simulink model "topology_comparison_eff"  (R2024b)
settings: Solver=ode23tb  StartTime=0.0  StopTime=4  MaxStep=1e-4  MinStep=1e-9  RelTol=1e-3
InitFcn:
  | sw_freq=60e3;
  | eff_rms_freq=sw_freq/10;
  | V_high=80;
  | 
  | L_ind=300e-6;
  | L_res=20e-3;
  | 
  | MOS_Ron=10e-3;
  | MOS_Vfw=1.2;
  | 
  | DIO_Vfw=0.9;
  | DIO_Ron=2e-3;
  | 
  | TRC_Res=5e-3;
  | 
  | sync_mode=1;
  | 
  | buck_p=0.02;
  | buck_i=0.8;
  | 
  | inter_bdc_p=0.02;
  | inter_bdc_i=0.9;
  | 
  | asym_bdc_p=0.02;
  | asym_bdc_i=1.1;
values from neighbouring files (symbols this model uses):
  runtime = 4    [compare_conv_eff.m]
  timestep = runtime/size(curr_range,2)    [compare_conv_eff.m]
undefined symbols (not defined in the file or in its folder): V_low
libraries: spsMeanLib x14, spsGroundLib x14, spsSeriesRLCBranchLib x14, spsMosfetLib x10, slpidlib x7, spsDCVoltageSourceLib x6, spsMultimeterLib x3, spsDiodeLib x2, embmathops x1, spsStairGeneratorLib x1, spspowerguiLib x1
(part 1 of 2)
settings Model: SimulationMode=rapid-accelerator  Creator=adamo  LastModifiedBy=adamo
settings DebuggingCC: MaskedZcDiagnostic=none  IgnoredZcDiagnostic=none
settings HardwareCC: ProdHWDeviceType=AMD->x86-64 (Windows64)
settings RTWCC: BuildConfiguration=Faster Runs  CheckMdlBeforeBuild=Error
settings GRTTargetCC: OptimizeReductions=on
settings SimscapeCC: SimscapeCompileComponentReuse=on  SimscapeCompileArtifactsDiskCache=on

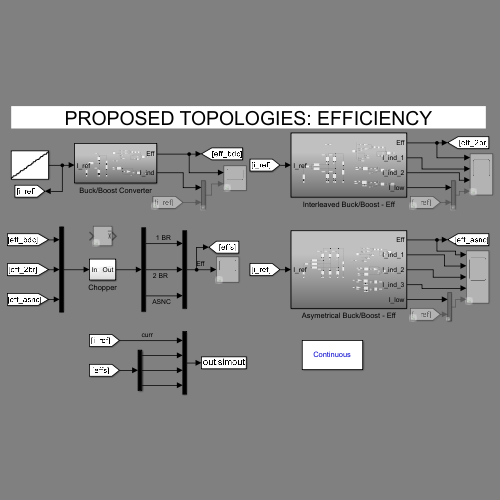
[thumbnail: Simulink's stored preview of the top-level diagram]
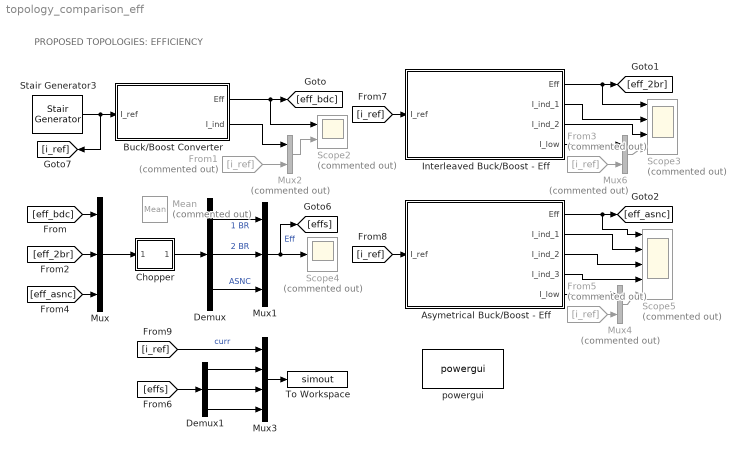
== system topology_comparison_eff ==
  note: PROPOSED TOPOLOGIES: EFFICIENCY
  Asymetrical Buck/Boost - Eff : Subsystem
  Buck/Boost Converter : Subsystem
  Chopper : Subsystem
  Demux : Demux  Outputs=3
  Demux1 : Demux  Outputs=3
  From1 : From  Commented=on  GotoTag=i_ref
  From3 : From  Commented=on  GotoTag=i_ref
  From5 : From  Commented=on  GotoTag=i_ref
  Interleaved Buck/Boost - Eff : Subsystem
  Mean : spsMeanLib/Mean  Commented=on  Freq=sw_freq/10  Vinit=0  Ts=0
  Mux : Mux  Inputs=3
  Mux1 : Mux  Inputs=3
  Mux2 : Mux  Commented=on  Inputs=2
  Mux3 : Mux
  Mux4 : Mux  Commented=on  Inputs=2
  Mux6 : Mux  Commented=on  Inputs=2
  Scope2 : Scope  Commented=on  NumInputPorts=2
  Scope3 : Scope  Commented=on  NumInputPorts=4
  Scope4 : Scope  Commented=on
  Scope5 : Scope  Commented=on  NumInputPorts=5
  Stair Generator3 : spsStairGeneratorLib/Stair Generator  t=[0:timestep:runtime-timestep]  e=curr_range  Ts=0
  To Workspace : ToWorkspace  VariableName=simout  SampleTime=-1
  powergui : spspowerguiLib/powergui  Priority=1  SimulationMode=Continuous  SampleTime=50e-6  frequency=60  Iterations=50  frequencyindice=0  Pbase=100e6  ErrMax=1e-4  UnitsV=kV  UnitsW=MW  buscounter=0  FunctionMessages=off  echomessages=off  EnableUseOfTLC=off  CurrentSourceSwitches=off  DisableSnubberDevices=on  DisableRonSwitches=off  DisableVfSwitches=off  DisplayEquations=off  AutomaticDiscreteSolvers=off  SolverType=Tustin/Backward Euler (TBE)  Interpol=off  ExternalGateDelay=off  methode=on  Ts=100  x0status=blocks  SPID=on  SwTol=0  HookPort=off  NonlinearTolerance=1e-4  nMaxIteration=100  ContinueOnMaxIteration=off  RestoreLinks=warning  ResistiveCurrentMeasurement=off  Frange=[0:2:500]  Ylog=off  Xlog=on  ShowGrid=off  save=off  variable=ZData  structure=0  ZoomFFT=off  StartTime=0.0  cycles=1  DisplayStyle=1  fundamental=60  FreqAxis=off  MaxFrequency=1000  frequencyindicesteady=1  RmsSteady=1  display=off
  wires:
  Stair Generator3/1 -> [i_ref], Buck/Boost Converter/1(I_ref)
  [i_ref] -> Interleaved Buck/Boost - Eff/1(I_ref)
  [i_ref] -> Asymetrical Buck/Boost - Eff/1(I_ref)
  Buck/Boost Converter/2(I_ind) -> Mux2/1
  Interleaved Buck/Boost - Eff/1(Eff) -> Scope3/1, [eff_2br]
  Interleaved Buck/Boost - Eff/3(I_ind_2) -> Scope3/3
  Interleaved Buck/Boost - Eff/2(I_ind_1) -> Scope3/2
  Asymetrical Buck/Boost - Eff/3(I_ind_2) -> Scope5/3
  Asymetrical Buck/Boost - Eff/4(I_ind_3) -> Scope5/4
  Buck/Boost Converter/1(Eff) -> Scope2/1, [eff_bdc]
  Asymetrical Buck/Boost - Eff/1(Eff) -> Scope5/1, [eff_asnc]
  [eff_bdc] -> Mux/1
  [eff_2br] -> Mux/2
  [eff_asnc] -> Mux/3
  Mux/1 -> Chopper/1(In1)
  Chopper/1(Out1) -> Demux/1
  Demux/1 -> Mux1/1  "1 BR"
  Demux/2 -> Mux1/2  "2 BR"
  Demux/3 -> Mux1/3  "ASNC"
  Mux1/1 -> [effs], Scope4/1  "Eff"
  [i_ref] -> Mux3/1  "curr"
  Mux3/1 -> To Workspace/1
  [effs] -> Demux1/1
  Demux1/1 -> Mux3/2
  Demux1/2 -> Mux3/3
  Demux1/3 -> Mux3/4
  Interleaved Buck/Boost - Eff/4(I_low) -> Mux6/1
  Asymetrical Buck/Boost - Eff/2(I_ind_1) -> Scope5/2
  From1/1 -> Mux2/2
  Mux2/1 -> Scope2/2
  From3/1 -> Mux6/2
  Mux6/1 -> Scope3/4
  From5/1 -> Mux4/2
  Asymetrical Buck/Boost - Eff/5(I_low) -> Mux4/1
  Mux4/1 -> Scope5/5

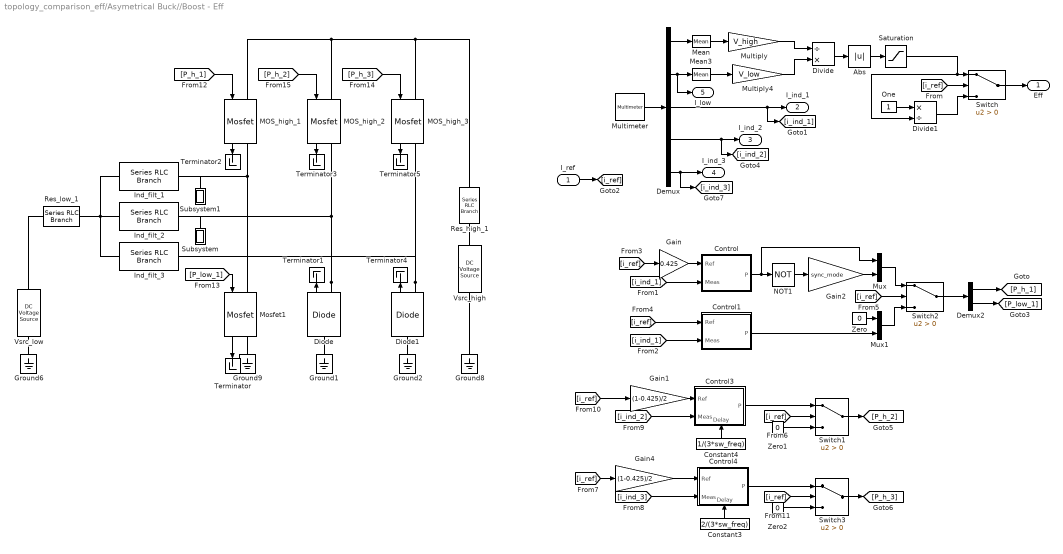
== system topology_comparison_eff/Asymetrical Buck//Boost - Eff ==
  I_ref : Inport
  Abs : Abs  SaturateOnIntegerOverflow=off
  Constant3 : Constant  Value=2/(3*sw_freq)
  Constant4 : Constant  Value=1/(3*sw_freq)
  Control : Subsystem
  Control1 : Subsystem
  Control3 : Subsystem
      settings: PortSchema="{\"entries\":[{\"content\":{\"sides\":[{\"content\":{\"connectorIds\":[\"In1\",\"In2\"]},\"type\":\"ConnectorPlacement.EquallySpacedRectSide\",\"uuid\":\"44975c06-6cb3-4b92-aa2e-c11b859d13e4\"},{\"content\":{\"connectorIds\":[\"Out1\"],\"side\":\"RIGHT\"},\"type\":\"ConnectorPlacement.EquallySpacedRectSide\",\"uuid\":\"ebdc9065-5b19-4aa7-8841-916fd82a5d31\"},{\"content\":{\"side\":\"TOP\"},\"type\":\"ConnectorPlacement.EquallySpacedRectSide\",\"uuid\":\"027925ea-888b-4bcf-b8a4-44694d0e275e\"},{\"content\":{\"connectorIds\":[\"In3\"],\"side\":\"BOTTOM\"},\"type\":\"ConnectorPlacement.EquallySpacedRectSide\",\"uuid\":\"415fb0af-dd9a-4309-9118-76332ed11379\"}]},\"type\":\"ConnectorPlacement.EquallySpacedConnector\",\"uuid\":\"3cd19595-535e-42c3-a0e6-40045bedee28\"}],\"packageUris\":[\"http://schema.mathworks.com/mf0/Connector/R2020b\"],\"version\":\"1.0\"}"
  Control4 : Subsystem
      settings: PortSchema="{\"entries\":[{\"content\":{\"sides\":[{\"content\":{\"connectorIds\":[\"In1\",\"In2\"]},\"type\":\"ConnectorPlacement.EquallySpacedRectSide\",\"uuid\":\"44975c06-6cb3-4b92-aa2e-c11b859d13e4\"},{\"content\":{\"connectorIds\":[\"Out1\"],\"side\":\"RIGHT\"},\"type\":\"ConnectorPlacement.EquallySpacedRectSide\",\"uuid\":\"ebdc9065-5b19-4aa7-8841-916fd82a5d31\"},{\"content\":{\"side\":\"TOP\"},\"type\":\"ConnectorPlacement.EquallySpacedRectSide\",\"uuid\":\"027925ea-888b-4bcf-b8a4-44694d0e275e\"},{\"content\":{\"connectorIds\":[\"In3\"],\"side\":\"BOTTOM\"},\"type\":\"ConnectorPlacement.EquallySpacedRectSide\",\"uuid\":\"9488b47a-c58c-42e9-bacd-7bb9f563b775\"}]},\"type\":\"ConnectorPlacement.EquallySpacedConnector\",\"uuid\":\"3cd19595-535e-42c3-a0e6-40045bedee28\"}],\"packageUris\":[\"http://schema.mathworks.com/mf0/Connector/R2020b\"],\"version\":\"1.0\"}"
  Demux : Demux  Outputs=5
  Demux2 : Demux  Outputs=2
  Diode : spsDiodeLib/Diode  Ron=DIO_Ron  Lon=0  Vf=DIO_Vfw  IC=0  UseSnubber=0  Rs=500  Cs=250e-9  Measurements=on
  Diode1 : spsDiodeLib/Diode  Ron=DIO_Ron  Lon=0  Vf=DIO_Vfw  IC=0  UseSnubber=0  Rs=500  Cs=250e-9  Measurements=on
  Divide : Product  Inputs=/*
  Divide1 : Product  Inputs=*/
  Gain : Gain  Gain=0.425
  Gain1 : Gain  Gain=(1-0.425)/2
  Gain2 : Gain  Gain=sync_mode  OutDataTypeStr=double
  Gain4 : Gain  Gain=(1-0.425)/2
  Ground{1..2,6,8..9} (5 alike) : spsGroundLib/Ground  LConnTagsString=a
  Ind_filt_1 : spsSeriesRLCBranchLib/Series RLC Branch  LConnTagsString=__new0  RConnTagsString=__new0  BranchType=RL  Resistance=L_res  Inductance=L_ind  SetiL0=off  InitialCurrent=0  Capacitance=1e-6  Setx0=off  InitialVoltage=0  Measurements=Branch current
  Ind_filt_2 : spsSeriesRLCBranchLib/Series RLC Branch  LConnTagsString=__new0  RConnTagsString=__new0  BranchType=RL  Resistance=L_res  Inductance=L_ind  SetiL0=off  InitialCurrent=0  Capacitance=1e-6  Setx0=off  InitialVoltage=0  Measurements=Branch current
  Ind_filt_3 : spsSeriesRLCBranchLib/Series RLC Branch  LConnTagsString=__new0  RConnTagsString=__new0  BranchType=RL  Resistance=L_res  Inductance=L_ind  SetiL0=off  InitialCurrent=0  Capacitance=1e-6  Setx0=off  InitialVoltage=0  Measurements=Branch current
  MOS_high_1 : spsMosfetLib/Mosfet  Ron=MOS_Ron  Lon=0  Rd=DIO_Ron  Vfd=MOS_Vfw  IC=0  Rs=1e5  Cs=inf  Measurements=on
  MOS_high_2 : spsMosfetLib/Mosfet  Ron=MOS_Ron  Lon=0  Rd=DIO_Ron  Vfd=MOS_Vfw  IC=0  Rs=1e5  Cs=inf  Measurements=on
  MOS_high_3 : spsMosfetLib/Mosfet  Ron=MOS_Ron  Lon=0  Rd=DIO_Ron  Vfd=MOS_Vfw  IC=0  Rs=1e5  Cs=inf  Measurements=on
  Mean : spsMeanLib/Mean  Freq=eff_rms_freq  Vinit=1  Ts=0
  Mean3 : spsMeanLib/Mean  Freq=eff_rms_freq  Vinit=1  Ts=0
  Mosfet1 : spsMosfetLib/Mosfet  Ron=MOS_Ron  Lon=0  Rd=DIO_Ron  Vfd=MOS_Vfw  IC=0  Rs=1e5  Cs=inf  Measurements=on
  Multimeter : spsMultimeterLib/Multimeter  L=12  sel=[4 5 1 2 3]  yselected={}  Gain=[1 1 1 1 1]  OutputType=Complex  PlotAtSimulationStop=off  PhasorSimulation=off
  Multiply : Gain  Gain=V_high
  Multiply4 : Gain  Gain=V_low
  Mux : Mux  Inputs=2
  Mux1 : Mux  Inputs=2
  NOT1 : Logic  Operator=NOT  IconShape=distinctive  AllPortsSameDT=off  OutDataTypeStr=boolean
  One : Constant  OutDataTypeStr=Inherit: Inherit via back propagation
  Res_high_1 : spsSeriesRLCBranchLib/Series RLC Branch  LConnTagsString=__new0  RConnTagsString=__new0  BranchType=R  Resistance=TRC_Res  Inductance=1e-3  SetiL0=off  InitialCurrent=0  Capacitance=1e-6  Setx0=off  InitialVoltage=0  Measurements=Branch current
  Res_low_1 : spsSeriesRLCBranchLib/Series RLC Branch  LConnTagsString=__new0  RConnTagsString=__new0  BranchType=R  Resistance=TRC_Res  Inductance=1e-3  SetiL0=off  InitialCurrent=0  Capacitance=1e-6  Setx0=off  InitialVoltage=0  Measurements=Branch current
  Saturation : Saturate  UpperLimit=0.9999  LowerLimit=0.4
  Subsystem : Subsystem
      settings: PortSchema="{\"entries\":[{\"content\":{\"sides\":[{\"content\":{},\"type\":\"ConnectorPlacement.EquallySpacedRectSide\",\"uuid\":\"333a472d-5660-403e-9749-9e5a485a4e51\"},{\"content\":{\"side\":\"RIGHT\"},\"type\":\"ConnectorPlacement.EquallySpacedRectSide\",\"uuid\":\"46e3a3df-9b43-4056-bf49-6d97e0ff375e\"},{\"content\":{\"connectorIds\":[\"LConn1\"],\"side\":\"TOP\"},\"type\":\"ConnectorPlacement.EquallySpacedRectSide\",\"uuid\":\"a9be43b9-3284-437d-b483-2a714199e3a2\"}]},\"type\":\"ConnectorPlacement.EquallySpacedConnector\",\"uuid\":\"6030dd83-63ea-4a67-9f73-95d000b3af89\"}],\"packageUris\":[\"http://schema.mathworks.com/mf0/Connector/R2020b\"],\"version\":\"1.0\"}"
  Subsystem1 : Subsystem
      settings: PortSchema="{\"entries\":[{\"content\":{\"sides\":[{\"content\":{},\"type\":\"ConnectorPlacement.EquallySpacedRectSide\",\"uuid\":\"333a472d-5660-403e-9749-9e5a485a4e51\"},{\"content\":{\"side\":\"RIGHT\"},\"type\":\"ConnectorPlacement.EquallySpacedRectSide\",\"uuid\":\"46e3a3df-9b43-4056-bf49-6d97e0ff375e\"},{\"content\":{\"connectorIds\":[\"LConn1\"],\"side\":\"TOP\"},\"type\":\"ConnectorPlacement.EquallySpacedRectSide\",\"uuid\":\"a9be43b9-3284-437d-b483-2a714199e3a2\"}]},\"type\":\"ConnectorPlacement.EquallySpacedConnector\",\"uuid\":\"6030dd83-63ea-4a67-9f73-95d000b3af89\"}],\"packageUris\":[\"http://schema.mathworks.com/mf0/Connector/R2020b\"],\"version\":\"1.0\"}"
  Switch{,1..3} (4 alike) : Switch  Criteria=u2 > Threshold  SaturateOnIntegerOverflow=off  InputSameDT=off
  Terminator{,1..5} (6 alike) : Terminator
  Vsrc_high : spsDCVoltageSourceLib/DC Voltage Source  Amplitude=V_high  Measurements=None
  Vsrc_low : spsDCVoltageSourceLib/DC Voltage Source  Amplitude=V_low  Measurements=None
  Zero : Constant  Value=0  OutDataTypeStr=Inherit: Inherit via back propagation
  Zero1 : Constant  Value=0  OutDataTypeStr=Inherit: Inherit via back propagation
  Zero2 : Constant  Value=0  OutDataTypeStr=Inherit: Inherit via back propagation
  Eff : Outport
  I_ind_1 : Outport  Port=2
  I_ind_2 : Outport  Port=3
  I_ind_3 : Outport  Port=4
  I_low : Outport  Port=5
  wires:
  [P_h_1] -> MOS_high_1/1
  MOS_high_1/1 -> Terminator2/1
  Mosfet1/1 -> Terminator/1
  [P_low_1] -> Mosfet1/1
  Diode/1 -> Terminator1/1
  MOS_high_2/1 -> Terminator3/1
  Diode1/1 -> Terminator4/1
  MOS_high_3/1 -> Terminator5/1
  [P_h_3] -> MOS_high_3/1
  Multimeter/1 -> Demux/1
  One/1 -> Divide1/1
  Mean/1 -> Multiply/1
  Divide1/1 -> Switch/3
  Saturation/1 -> Divide1/2, Switch/1
  Divide/1 -> Abs/1
  Switch/1 -> Eff/1
  Abs/1 -> Saturation/1
  Control/1(P) -> Mux/1, NOT1/1
  [i_ref] -> Gain/1
  Switch2/1 -> Demux2/1
  Mux/1 -> Switch2/1
  [i_ind_1] -> Control/2(Meas)
  Demux2/2 -> [P_low_1]
  Demux2/1 -> [P_h_1]
  Gain2/1 -> Mux/2
  [i_ref] -> Switch2/2
  I_ref/1 -> [i_ref]
  [i_ref] -> Switch/2
  NOT1/1 -> Gain2/1
  [P_h_2] -> MOS_high_2/1
  Gain/1 -> Control/1(Ref)
  [i_ref] -> Control1/1(Ref)
  [i_ind_1] -> Control1/2(Meas)
  Control1/1(P) -> Mux1/2
  Mean3/1 -> Multiply4/1
  Demux/1 -> Mean/1
  Demux/2 -> I_low/1, Mean3/1
  Demux/5 -> [i_ind_3], I_ind_3/1
  Demux/4 -> [i_ind_2], I_ind_2/1
  Demux/3 -> I_ind_1/1, [i_ind_1]
  Multiply4/1 -> Divide/2
  Multiply/1 -> Divide/1
  Mux1/1 -> Switch2/3
  Zero/1 -> Mux1/1
  Constant4/1 -> Control3/3(Delay)
  Constant3/1 -> Control4/3(Delay)
  [i_ref] -> Gain1/1
  Gain1/1 -> Control3/1(Ref)
  [i_ind_2] -> Control3/2(Meas)
  Control3/1(P) -> Switch1/1
  Switch1/1 -> [P_h_2]
  Zero1/1 -> Switch1/3
  [i_ref] -> Switch1/2
  [i_ind_3] -> Control4/2(Meas)
  [i_ref] -> Gain4/1
  Gain4/1 -> Control4/1(Ref)
  [i_ref] -> Switch3/2
  Control4/1(P) -> Switch3/1
  Switch3/1 -> [P_h_3]
  Zero2/1 -> Switch3/3
  connections:
  Diode/RConn1 -- Ind_filt_2/LConn1 -- Subsystem/LConn1 -- MOS_high_2/RConn1
  MOS_high_1/RConn1 -- Subsystem1/LConn1 -- Ind_filt_1/LConn1 -- Mosfet1/LConn1
  Ground8/LConn1 -- Vsrc_high/LConn1
  Mosfet1/RConn1 -- Ground9/LConn1
  Ground6/LConn1 -- Vsrc_low/LConn1
  Diode/LConn1 -- Ground1/LConn1
  Diode1/RConn1 -- Ind_filt_3/LConn1 -- MOS_high_3/RConn1
  Diode1/LConn1 -- Ground2/LConn1
  Res_low_1/RConn1 -- Vsrc_low/RConn1
  Res_high_1/LConn1 -- Vsrc_high/RConn1
  Ind_filt_2/RConn1 -- Res_low_1/LConn1 -- Ind_filt_3/RConn1 -- Ind_filt_1/RConn1
  Res_high_1/RConn1 -- MOS_high_1/LConn1 -- MOS_high_2/LConn1 -- MOS_high_3/LConn1

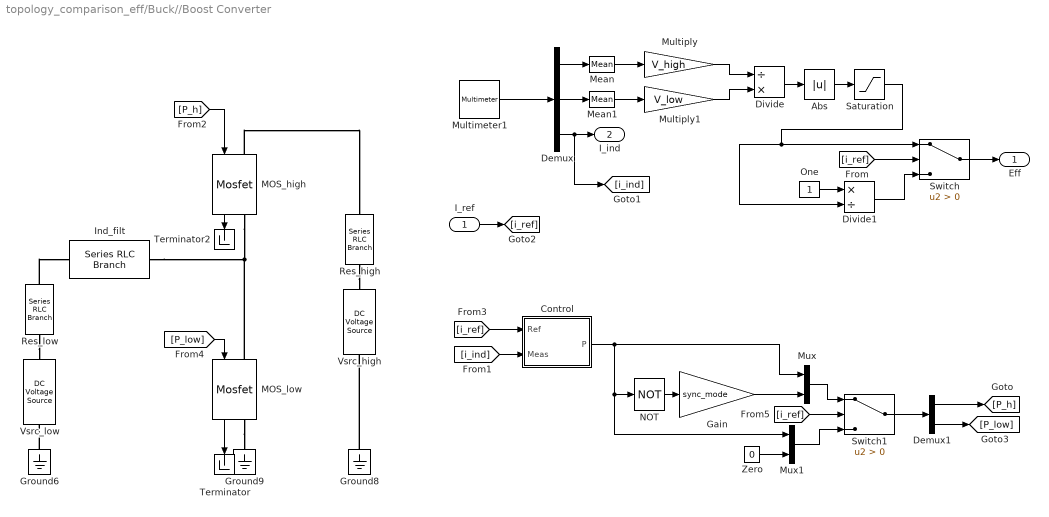
== system topology_comparison_eff/Buck//Boost Converter ==
  I_ref : Inport
  Abs : Abs  SaturateOnIntegerOverflow=off
  Control : Subsystem
  Demux : Demux  Outputs=3
  Demux1 : Demux  Outputs=2
  Divide : Product  Inputs=/*
  Divide1 : Product  Inputs=*/
  Gain : Gain  Gain=sync_mode  OutDataTypeStr=double
  Ground6 : spsGroundLib/Ground  LConnTagsString=a
  Ground8 : spsGroundLib/Ground  LConnTagsString=a
  Ground9 : spsGroundLib/Ground  LConnTagsString=a
  Ind_filt : spsSeriesRLCBranchLib/Series RLC Branch  LConnTagsString=__new0  RConnTagsString=__new0  BranchType=RL  Resistance=L_res  Inductance=L_ind  SetiL0=off  InitialCurrent=0  Capacitance=1e-6  Setx0=off  InitialVoltage=0  Measurements=Branch current
  MOS_high : spsMosfetLib/Mosfet  Ron=MOS_Ron  Lon=0  Rd=DIO_Ron  Vfd=MOS_Vfw  IC=0  Rs=1e5  Cs=inf  Measurements=on
  MOS_low : spsMosfetLib/Mosfet  Ron=MOS_Ron  Lon=0  Rd=DIO_Ron  Vfd=MOS_Vfw  IC=0  Rs=1e5  Cs=inf  Measurements=on
  Mean : spsMeanLib/Mean  Freq=eff_rms_freq  Vinit=1  Ts=0
  Mean1 : spsMeanLib/Mean  Freq=eff_rms_freq  Vinit=1  Ts=0
  Multimeter1 : spsMultimeterLib/Multimeter  L=12  sel=[7 8 6]  yselected={}  Gain=[1 1 1]  OutputType=Complex  PlotAtSimulationStop=off  PhasorSimulation=off
  Multiply : Gain  Gain=V_high
  Multiply1 : Gain  Gain=V_low
  Mux : Mux  Inputs=2
  Mux1 : Mux  Inputs=2
  NOT : Logic  Operator=NOT  IconShape=distinctive  AllPortsSameDT=off  OutDataTypeStr=boolean
  One : Constant  OutDataTypeStr=Inherit: Inherit via back propagation
  Res_high : spsSeriesRLCBranchLib/Series RLC Branch  LConnTagsString=__new0  RConnTagsString=__new0  BranchType=R  Resistance=TRC_Res  Inductance=1e-3  SetiL0=off  InitialCurrent=0  Capacitance=1e-6  Setx0=off  InitialVoltage=0  Measurements=Branch current
  Res_low : spsSeriesRLCBranchLib/Series RLC Branch  LConnTagsString=__new0  RConnTagsString=__new0  BranchType=R  Resistance=TRC_Res  Inductance=1e-3  SetiL0=off  InitialCurrent=0  Capacitance=1e-6  Setx0=off  InitialVoltage=0  Measurements=Branch current
  Saturation : Saturate  UpperLimit=0.9999  LowerLimit=0.4
  Switch : Switch  Criteria=u2 > Threshold  SaturateOnIntegerOverflow=off  InputSameDT=off
  Switch1 : Switch  Criteria=u2 > Threshold  SaturateOnIntegerOverflow=off  InputSameDT=off
  Terminator : Terminator
  Terminator2 : Terminator
  Vsrc_high : spsDCVoltageSourceLib/DC Voltage Source  Amplitude=V_high  Measurements=None
  Vsrc_low : spsDCVoltageSourceLib/DC Voltage Source  Amplitude=V_low  Measurements=None
  Zero : Constant  Value=0  OutDataTypeStr=Inherit: Inherit via back propagation
  Eff : Outport
  I_ind : Outport  Port=2
  wires:
  MOS_low/1 -> Terminator/1
  MOS_high/1 -> Terminator2/1
  [P_h] -> MOS_high/1
  [P_low] -> MOS_low/1
  Multiply/1 -> Divide/1
  Demux/1 -> Mean/1
  Saturation/1 -> Divide1/2, Switch/1
  Multiply1/1 -> Divide/2
  Mean/1 -> Multiply/1
  Multimeter1/1 -> Demux/1
  Demux/2 -> Mean1/1
  Mean1/1 -> Multiply1/1
  One/1 -> Divide1/1
  Divide1/1 -> Switch/3
  Switch/1 -> Eff/1
  Divide/1 -> Abs/1
  Demux/3 -> [i_ind], I_ind/1
  Control/1(P) -> Mux1/1, NOT/1, Mux/1
  I_ref/1 -> [i_ref]
  [i_ref] -> Switch/2
  [i_ind] -> Control/2(Meas)
  [i_ref] -> Control/1(Ref)
  NOT/1 -> Gain/1
  Abs/1 -> Saturation/1
  [i_ref] -> Switch1/2
  Mux/1 -> Switch1/1
  Switch1/1 -> Demux1/1
  Demux1/1 -> [P_h]
  Demux1/2 -> [P_low]
  Zero/1 -> Mux1/2
  Mux1/1 -> Switch1/3
  Gain/1 -> Mux/2
  connections:
  MOS_high/LConn1 -- Res_high/RConn1
  MOS_low/RConn1 -- Ground9/LConn1
  MOS_high/RConn1 -- Ind_filt/LConn1 -- MOS_low/LConn1
  Ground8/LConn1 -- Vsrc_high/LConn1
  Ground6/LConn1 -- Vsrc_low/LConn1
  Res_low/LConn1 -- Ind_filt/RConn1
  Res_high/LConn1 -- Vsrc_high/RConn1
  Res_low/RConn1 -- Vsrc_low/RConn1

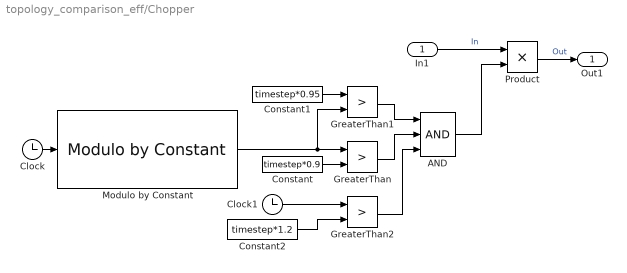
== system topology_comparison_eff/Chopper ==
  In1 : Inport
  AND : Logic  Inputs=3  IconShape=distinctive  AllPortsSameDT=off  OutDataTypeStr=boolean
  Clock : Clock
  Clock1 : Clock
  Constant : Constant  Value=timestep*0.9
  Constant1 : Constant  Value=timestep*0.95
  Constant2 : Constant  Value=timestep*1.2
  GreaterThan : RelationalOperator  Operator=>  OutDataTypeStr=boolean  RndMeth=Simplest  InputSameDT=off
  GreaterThan1 : RelationalOperator  Operator=>  OutDataTypeStr=boolean  RndMeth=Simplest  InputSameDT=off
  GreaterThan2 : RelationalOperator  Operator=>  OutDataTypeStr=boolean  RndMeth=Simplest  InputSameDT=off
  Modulo by Constant : embmathops/Modulo by Constant  Denominator=timestep  SimulateUsing=Code generation
  Product : Product
  Out1 : Outport
  wires:
  Clock/1 -> Modulo by Constant/1
  Constant/1 -> GreaterThan/2
  GreaterThan1/1 -> AND/1
  GreaterThan/1 -> AND/2
  AND/1 -> Product/2
  Modulo by Constant/1 -> GreaterThan1/2, GreaterThan/1
  Constant1/1 -> GreaterThan1/1
  In1/1 -> Product/1  "In"
  Product/1 -> Out1/1  "Out"
  Clock1/1 -> GreaterThan2/1
  GreaterThan2/1 -> AND/3
  Constant2/1 -> GreaterThan2/2

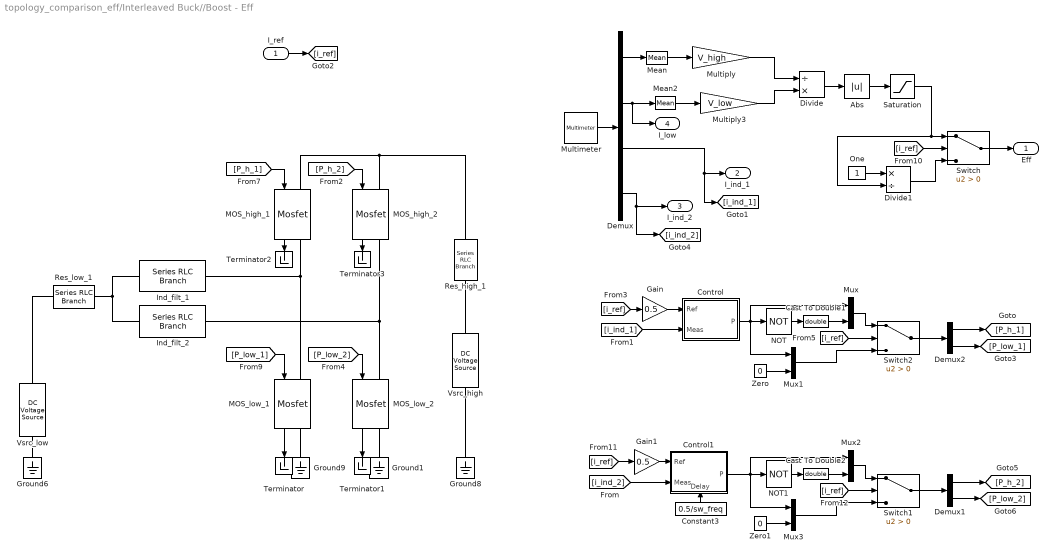
== system topology_comparison_eff/Interleaved Buck//Boost - Eff ==
  I_ref : Inport
  Abs : Abs  SaturateOnIntegerOverflow=off
  Cast To Double1 : DataTypeConversion  OutDataTypeStr=double  SaturateOnIntegerOverflow=off  RndMeth=Floor
  Cast To Double2 : DataTypeConversion  OutDataTypeStr=double  SaturateOnIntegerOverflow=off  RndMeth=Floor
  Constant3 : Constant  Value=0.5/sw_freq
  Control : Subsystem
  Control1 : Subsystem
      settings: PortSchema="{\"entries\":[{\"content\":{\"sides\":[{\"content\":{\"connectorIds\":[\"In1\",\"In2\"]},\"type\":\"ConnectorPlacement.EquallySpacedRectSide\",\"uuid\":\"44975c06-6cb3-4b92-aa2e-c11b859d13e4\"},{\"content\":{\"connectorIds\":[\"Out1\"],\"side\":\"RIGHT\"},\"type\":\"ConnectorPlacement.EquallySpacedRectSide\",\"uuid\":\"ebdc9065-5b19-4aa7-8841-916fd82a5d31\"},{\"content\":{\"side\":\"TOP\"},\"type\":\"ConnectorPlacement.EquallySpacedRectSide\",\"uuid\":\"027925ea-888b-4bcf-b8a4-44694d0e275e\"},{\"content\":{\"connectorIds\":[\"In3\"],\"side\":\"BOTTOM\"},\"type\":\"ConnectorPlacement.EquallySpacedRectSide\",\"uuid\":\"4b21ce2f-6f21-43cd-b77f-3dbeff0cb919\"}]},\"type\":\"ConnectorPlacement.EquallySpacedConnector\",\"uuid\":\"3cd19595-535e-42c3-a0e6-40045bedee28\"}],\"packageUris\":[\"http://schema.mathworks.com/mf0/Connector/R2020b\"],\"version\":\"1.0\"}"
  Demux : Demux
  Demux1 : Demux  Outputs=2
  Demux2 : Demux  Outputs=2
  Divide : Product  Inputs=/*
  Divide1 : Product  Inputs=*/
  Gain : Gain  Gain=0.5
  Gain1 : Gain  Gain=0.5
  Ground{1,6,8..9} (4 alike) : spsGroundLib/Ground  LConnTagsString=a
  Ind_filt_1 : spsSeriesRLCBranchLib/Series RLC Branch  LConnTagsString=__new0  RConnTagsString=__new0  BranchType=RL  Resistance=L_res*2/3  Inductance=L_ind  SetiL0=off  InitialCurrent=0  Capacitance=1e-6  Setx0=off  InitialVoltage=0  Measurements=Branch current
  Ind_filt_2 : spsSeriesRLCBranchLib/Series RLC Branch  LConnTagsString=__new0  RConnTagsString=__new0  BranchType=RL  Resistance=L_res*2/3  Inductance=L_ind  SetiL0=off  InitialCurrent=0  Capacitance=1e-6  Setx0=off  InitialVoltage=0  Measurements=Branch current
  MOS_high_1 : spsMosfetLib/Mosfet  Ron=MOS_Ron  Lon=0  Rd=DIO_Ron  Vfd=MOS_Vfw  IC=0  Rs=1e5  Cs=inf  Measurements=on
  MOS_high_2 : spsMosfetLib/Mosfet  Ron=MOS_Ron  Lon=0  Rd=DIO_Ron  Vfd=MOS_Vfw  IC=0  Rs=1e5  Cs=inf  Measurements=on
  MOS_low_1 : spsMosfetLib/Mosfet  Ron=MOS_Ron  Lon=0  Rd=DIO_Ron  Vfd=MOS_Vfw  IC=0  Rs=1e5  Cs=inf  Measurements=on
  MOS_low_2 : spsMosfetLib/Mosfet  Ron=MOS_Ron  Lon=0  Rd=DIO_Ron  Vfd=MOS_Vfw  IC=0  Rs=1e5  Cs=inf  Measurements=on
  Mean : spsMeanLib/Mean  Freq=eff_rms_freq  Vinit=1  Ts=0
  Mean2 : spsMeanLib/Mean  Freq=eff_rms_freq  Vinit=1  Ts=0
  Multimeter : spsMultimeterLib/Multimeter  L=12  sel=[11 12 9 10]  yselected={}  Gain=[1 1 1 1]  OutputType=Complex  PlotAtSimulationStop=off  PhasorSimulation=off
  Multiply : Gain  Gain=V_high
  Multiply3 : Gain  Gain=V_low
  Mux{,1..3} (4 alike) : Mux  Inputs=2
  NOT : Logic  Operator=NOT  IconShape=distinctive  AllPortsSameDT=off  OutDataTypeStr=boolean
  NOT1 : Logic  Operator=NOT  IconShape=distinctive  AllPortsSameDT=off  OutDataTypeStr=boolean
  One : Constant  OutDataTypeStr=Inherit: Inherit via back propagation
  Res_high_1 : spsSeriesRLCBranchLib/Series RLC Branch  LConnTagsString=__new0  RConnTagsString=__new0  BranchType=R  Resistance=TRC_Res  Inductance=1e-3  SetiL0=off  InitialCurrent=0  Capacitance=1e-6  Setx0=off  InitialVoltage=0  Measurements=Branch current
  Res_low_1 : spsSeriesRLCBranchLib/Series RLC Branch  LConnTagsString=__new0  RConnTagsString=__new0  BranchType=R  Resistance=TRC_Res  Inductance=1e-3  SetiL0=off  InitialCurrent=0  Capacitance=1e-6  Setx0=off  InitialVoltage=0  Measurements=Branch current
  Saturation : Saturate  UpperLimit=0.9999  LowerLimit=0.4
  Switch : Switch  Criteria=u2 > Threshold  SaturateOnIntegerOverflow=off  InputSameDT=off
  Switch1 : Switch  Criteria=u2 > Threshold  SaturateOnIntegerOverflow=off  InputSameDT=off
  Switch2 : Switch  Criteria=u2 > Threshold  SaturateOnIntegerOverflow=off  InputSameDT=off
  Terminator{,1..3} (4 alike) : Terminator
  Vsrc_high : spsDCVoltageSourceLib/DC Voltage Source  Amplitude=V_high  Measurements=None
  Vsrc_low : spsDCVoltageSourceLib/DC Voltage Source  Amplitude=V_low  Measurements=None
  Zero : Constant  Value=0  OutDataTypeStr=Inherit: Inherit via back propagation
  Zero1 : Constant  Value=0  OutDataTypeStr=Inherit: Inherit via back propagation
  Eff : Outport
  I_ind_1 : Outport  Port=2
  I_ind_2 : Outport  Port=3
  I_low : Outport  Port=4
  wires:
  [P_h_1] -> MOS_high_1/1
  [P_low_2] -> MOS_low_2/1
  MOS_high_1/1 -> Terminator2/1
  MOS_low_1/1 -> Terminator/1
  MOS_low_2/1 -> Terminator1/1
  MOS_high_2/1 -> Terminator3/1
  [P_low_1] -> MOS_low_1/1
  Divide/1 -> Abs/1
  Saturation/1 -> Divide1/2, Switch/1
  Divide1/1 -> Switch/3
  One/1 -> Divide1/1
  Multimeter/1 -> Demux/1
  Demux/1 -> Mean/1
  Mean/1 -> Multiply/1
  Switch/1 -> Eff/1
  Demux/3 -> I_ind_1/1, [i_ind_1]
  Demux/4 -> I_ind_2/1, [i_ind_2]
  Abs/1 -> Saturation/1
  [i_ref] -> Switch2/2
  NOT/1 -> Cast To Double1/1
  I_ref/1 -> [i_ref]
  Zero/1 -> Mux1/2
  Demux2/1 -> [P_h_1]
  Demux2/2 -> [P_low_1]
  [i_ref] -> Gain/1
  Mux/1 -> Switch2/1
  Switch2/1 -> Demux2/1
  [i_ind_1] -> Control/2(Meas)
  [i_ref] -> Switch/2
  Mux1/1 -> Switch2/3
  Cast To Double1/1 -> Mux/2
  Gain/1 -> Control/1(Ref)
  Control/1(P) -> Mux/1, Mux1/1, NOT/1
  [P_h_2] -> MOS_high_2/1
  Mean2/1 -> Multiply3/1
  Demux/2 -> I_low/1, Mean2/1
  Multiply3/1 -> Divide/2
  Multiply/1 -> Divide/1
  Constant3/1 -> Control1/3(Delay)
  Gain1/1 -> Control1/1(Ref)
  [i_ind_2] -> Control1/2(Meas)
  [i_ref] -> Gain1/1
  [i_ref] -> Switch1/2
  Zero1/1 -> Mux3/2
  Mux2/1 -> Switch1/1
  Mux3/1 -> Switch1/3
  Demux1/2 -> [P_low_2]
  Demux1/1 -> [P_h_2]
  Cast To Double2/1 -> Mux2/2
  NOT1/1 -> Cast To Double2/1
  Control1/1(P) -> Mux2/1, Mux3/1, NOT1/1
  Switch1/1 -> Demux1/1
  connections:
  MOS_high_2/RConn1 -- Ind_filt_2/LConn1 -- MOS_low_2/LConn1
  MOS_high_1/RConn1 -- Ind_filt_1/LConn1 -- MOS_low_1/LConn1
  Ind_filt_2/RConn1 -- Res_low_1/LConn1 -- Ind_filt_1/RConn1
  Ground8/LConn1 -- Vsrc_high/LConn1
  MOS_low_1/RConn1 -- Ground9/LConn1
  Ground6/LConn1 -- Vsrc_low/LConn1
  MOS_low_2/RConn1 -- Ground1/LConn1
  Res_high_1/LConn1 -- Vsrc_high/RConn1
  Res_low_1/RConn1 -- Vsrc_low/RConn1
  Res_high_1/RConn1 -- MOS_high_1/LConn1 -- MOS_high_2/LConn1

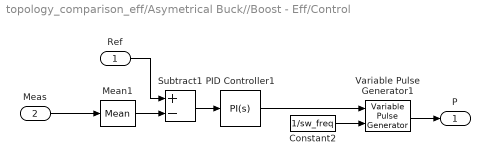
== system topology_comparison_eff/Asymetrical Buck//Boost - Eff/Control ==
  Ref : Inport
  Meas : Inport  Port=2
  Constant2 : Constant  Value=1/sw_freq
  Mean1 : spsMeanLib/Mean  Freq=sw_freq/10  Vinit=0  Ts=0
  PID Controller1 : slpidlib/PID Controller  Controller=PI  Form=Parallel  TimeDomain=Continuous-time  UseExternalTs=off  SampleTime=-1  IntegratorMethod=Forward Euler  FilterMethod=Forward Euler  ControllerParametersSource=internal  P=asym_bdc_p  I=asym_bdc_i  UseKiTs=on  D=0  UseExternalDerivativeSource=off  N=100  UseFilter=on  TunerSelectOption=Transfer Function Based (PID Tuner App)  InitialConditionSource=internal  InitialConditionForIntegrator=0.16  InitialConditionForFilter=0.1  DifferentiatorICPrevScaledInput=0  ExternalReset=none  TrackingMode=off  Kt=1  LimitOutput=on  SatLimitsSource=internal  UpperSaturationLimit=1  LowerSaturationLimit=0.01  LinearizeAsGain=on  AntiWindupMode=none  Kb=1  LimitIntegrator=off  UpperIntegratorSaturationLimit=inf  LowerIntegratorSaturationLimit=-inf  POutMin=[]  POutMax=[]  IOutMin=[]  IOutMax=[]  DOutMin=[]  DOutMax=[]  NOutMin=[]  NOutMax=[]  SumOutMin=[]  SumOutMax=[]  SaturationOutMin=[]  SaturationOutMax=[]  PParamMin=[]  PParamMax=[]  IParamMin=[]  IParamMax=[]  DParamMin=[]  DParamMax=[]  NParamMin=[]  NParamMax=[]  KbParamMin=[]  KbParamMax=[]  KtParamMin=[]  KtParamMax=[]  KbOutMin=[]  KbOutMax=[]  KtOutMin=[]  KtOutMax=[]  IntegratorOutMin=[]  IntegratorOutMax=[]  FilterOutMin=[]  FilterOutMax=[]  SumI1OutMin=[]  SumI1OutMax=[]  SumI2OutMin=[]  SumI2OutMax=[]  SumI3OutMin=[]  SumI3OutMax=[]  SumI4OutMin=[]  SumI4OutMax=[]  SumDOutMin=[]  SumDOutMax=[]  DifferentiatorOutMin=[]  DifferentiatorOutMax=[]  FilterDiffOutCoefMin=[]  FilterDiffOutCoefMax=[]  ReciprocalOutMin=[]  ReciprocalOutMax=[]  SumDenOutMin=[]  SumDenOutMax=[]  SumNumOutMin=[]  SumNumOutMax=[]  DivideOutMin=[]  DivideOutMax=[]  UdiffTsProdOutMin=[]  UdiffTsProdOutMax=[]  NTsProdOutMin=[]  NTsProdOutMax=[]  UintegralTsProdOutMin=[]  UintegralTsProdOutMax=[]  UngainTsProdOutMin=[]  UngainTsProdOutMax=[]  ClampingZeroOutDataTypeStr=Inherit: Inherit via back propagation  ClampingZeroOutMin=[]  ClampingZeroOutMax=[]  FilterDenConstantOutDataTypeStr=Inherit: Inherit via back propagation  FilterDenConstantOutMin=[]  FilterDenConstantOutMax=[]  PCopyOutDataTypeStr=Inherit: Inherit via back propagation  PCopyOutMin=[]  PCopyOutMax=[]  NCopyOutDataTypeStr=Inherit: Inherit via back propagation  NCopyOutMin=[]  NCopyOutMax=[]  IntegratorContinuousStateAttributes=''  IntegratorStateMustResolveToSignalObject=off  IntegratorRTWStateStorageClass=Auto  FilterContinuousStateAttributes=''  FilterStateMustResolveToSignalObject=off  FilterRTWStateStorageClass=Auto  ParallelPVariant=InternalParameters  IdealPVariant=Disabled  IVariant=InternalParameters  DVariant=Disabled  IntegratorVariant=Continuous  SatVariant=Enabled  AWVariant=Passthrough  PCopyVariant=Disabled  TRVariant=Disabled  FdbkBlocksVariant=Forward  IdealPFdbkVariant=Disabled  SatFdbkVariant=Disabled  DerivativeFilterVariant=Disabled  NVariant=Disabled  NCopyVariant=Disabled_SignalSpec  FilterICVariant=Disabled  IntegratorICVariant=InternalICs  ExternalResetVariant=Disabled  TRSumVariant=Passthrough  SumFdbkVariant=Disabled  SumVariant=Sum_PI  TsampFilterVariant=InternalTs  TsampNgainVariant=Passthrough  TsampIntegralVariant=Disabled_SignalSpec  ExternalSaturationOutDataTypeStr=Inherit: Same as second input  DerivativeSourceVariant=Disabled  PreIntVariant=InternalPreInt
  Subtract1 : Sum  Inputs=+-
  Variable Pulse Generator1 : VariablePulseGenerator  AllowZeroPulseWidth=on  SampleTime=0.1
  P : Outport
  wires:
  Meas/1 -> Mean1/1
  PID Controller1/1 -> Variable Pulse Generator1/1
  Constant2/1 -> Variable Pulse Generator1/2
  Mean1/1 -> Subtract1/2
  Subtract1/1 -> PID Controller1/1
  Variable Pulse Generator1/1 -> P/1
  Ref/1 -> Subtract1/1

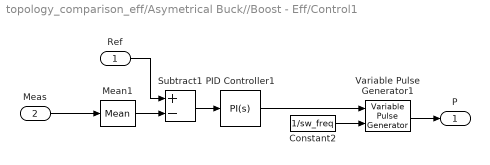
== system topology_comparison_eff/Asymetrical Buck//Boost - Eff/Control1 ==
  Ref : Inport
  Meas : Inport  Port=2
  Constant2 : Constant  Value=1/sw_freq
  Mean1 : spsMeanLib/Mean  Freq=sw_freq/10  Vinit=0  Ts=0
  PID Controller1 : slpidlib/PID Controller  Controller=PI  Form=Parallel  TimeDomain=Continuous-time  UseExternalTs=off  SampleTime=-1  IntegratorMethod=Forward Euler  FilterMethod=Forward Euler  ControllerParametersSource=internal  P=asym_bdc_p  I=asym_bdc_i  UseKiTs=on  D=0  UseExternalDerivativeSource=off  N=100  UseFilter=on  TunerSelectOption=Transfer Function Based (PID Tuner App)  InitialConditionSource=internal  InitialConditionForIntegrator=0  InitialConditionForFilter=0  DifferentiatorICPrevScaledInput=0  ExternalReset=none  TrackingMode=off  Kt=1  LimitOutput=on  SatLimitsSource=internal  UpperSaturationLimit=1  LowerSaturationLimit=0  LinearizeAsGain=on  AntiWindupMode=none  Kb=1  LimitIntegrator=off  UpperIntegratorSaturationLimit=inf  LowerIntegratorSaturationLimit=-inf  POutMin=[]  POutMax=[]  IOutMin=[]  IOutMax=[]  DOutMin=[]  DOutMax=[]  NOutMin=[]  NOutMax=[]  SumOutMin=[]  SumOutMax=[]  SaturationOutMin=[]  SaturationOutMax=[]  PParamMin=[]  PParamMax=[]  IParamMin=[]  IParamMax=[]  DParamMin=[]  DParamMax=[]  NParamMin=[]  NParamMax=[]  KbParamMin=[]  KbParamMax=[]  KtParamMin=[]  KtParamMax=[]  KbOutMin=[]  KbOutMax=[]  KtOutMin=[]  KtOutMax=[]  IntegratorOutMin=[]  IntegratorOutMax=[]  FilterOutMin=[]  FilterOutMax=[]  SumI1OutMin=[]  SumI1OutMax=[]  SumI2OutMin=[]  SumI2OutMax=[]  SumI3OutMin=[]  SumI3OutMax=[]  SumI4OutMin=[]  SumI4OutMax=[]  SumDOutMin=[]  SumDOutMax=[]  DifferentiatorOutMin=[]  DifferentiatorOutMax=[]  FilterDiffOutCoefMin=[]  FilterDiffOutCoefMax=[]  ReciprocalOutMin=[]  ReciprocalOutMax=[]  SumDenOutMin=[]  SumDenOutMax=[]  SumNumOutMin=[]  SumNumOutMax=[]  DivideOutMin=[]  DivideOutMax=[]  UdiffTsProdOutMin=[]  UdiffTsProdOutMax=[]  NTsProdOutMin=[]  NTsProdOutMax=[]  UintegralTsProdOutMin=[]  UintegralTsProdOutMax=[]  UngainTsProdOutMin=[]  UngainTsProdOutMax=[]  ClampingZeroOutDataTypeStr=Inherit: Inherit via back propagation  ClampingZeroOutMin=[]  ClampingZeroOutMax=[]  FilterDenConstantOutDataTypeStr=Inherit: Inherit via back propagation  FilterDenConstantOutMin=[]  FilterDenConstantOutMax=[]  PCopyOutDataTypeStr=Inherit: Inherit via back propagation  PCopyOutMin=[]  PCopyOutMax=[]  NCopyOutDataTypeStr=Inherit: Inherit via back propagation  NCopyOutMin=[]  NCopyOutMax=[]  IntegratorContinuousStateAttributes=''  IntegratorStateMustResolveToSignalObject=off  IntegratorRTWStateStorageClass=Auto  FilterContinuousStateAttributes=''  FilterStateMustResolveToSignalObject=off  FilterRTWStateStorageClass=Auto  ParallelPVariant=InternalParameters  IdealPVariant=Disabled  IVariant=InternalParameters  DVariant=Disabled  IntegratorVariant=Continuous  SatVariant=Enabled  AWVariant=Passthrough  PCopyVariant=Disabled  TRVariant=Disabled  FdbkBlocksVariant=Forward  IdealPFdbkVariant=Disabled  SatFdbkVariant=Disabled  DerivativeFilterVariant=Disabled  NVariant=Disabled  NCopyVariant=Disabled_SignalSpec  FilterICVariant=Disabled  IntegratorICVariant=InternalICs  ExternalResetVariant=Disabled  TRSumVariant=Passthrough  SumFdbkVariant=Disabled  SumVariant=Sum_PI  TsampFilterVariant=InternalTs  TsampNgainVariant=Passthrough  TsampIntegralVariant=Disabled_SignalSpec  ExternalSaturationOutDataTypeStr=Inherit: Same as second input  DerivativeSourceVariant=Disabled  PreIntVariant=InternalPreInt
  Subtract1 : Sum  Inputs=+-
  Variable Pulse Generator1 : VariablePulseGenerator  AllowZeroPulseWidth=on  SampleTime=0.1
  P : Outport
  wires:
  Meas/1 -> Mean1/1
  PID Controller1/1 -> Variable Pulse Generator1/1
  Constant2/1 -> Variable Pulse Generator1/2
  Mean1/1 -> Subtract1/2
  Subtract1/1 -> PID Controller1/1
  Variable Pulse Generator1/1 -> P/1
  Ref/1 -> Subtract1/1

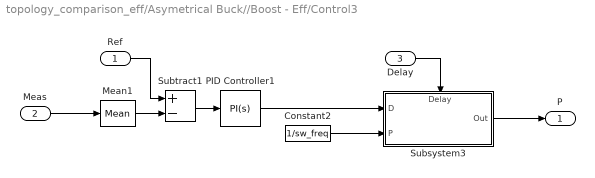
== system topology_comparison_eff/Asymetrical Buck//Boost - Eff/Control3 ==
  Ref : Inport
  Meas : Inport  Port=2
  Delay : Inport  Port=3
  Constant2 : Constant  Value=1/sw_freq
  Mean1 : spsMeanLib/Mean  Freq=sw_freq/10  Vinit=0  Ts=0
  PID Controller1 : slpidlib/PID Controller  Controller=PI  Form=Parallel  TimeDomain=Continuous-time  UseExternalTs=off  SampleTime=-1  IntegratorMethod=Forward Euler  FilterMethod=Forward Euler  ControllerParametersSource=internal  P=asym_bdc_p  I=asym_bdc_i  UseKiTs=on  D=0  UseExternalDerivativeSource=off  N=100  UseFilter=on  TunerSelectOption=Transfer Function Based (PID Tuner App)  InitialConditionSource=internal  InitialConditionForIntegrator=0.18  InitialConditionForFilter=0.1  DifferentiatorICPrevScaledInput=0  ExternalReset=none  TrackingMode=off  Kt=1  LimitOutput=on  SatLimitsSource=internal  UpperSaturationLimit=1  LowerSaturationLimit=0.01  LinearizeAsGain=on  AntiWindupMode=none  Kb=1  LimitIntegrator=off  UpperIntegratorSaturationLimit=inf  LowerIntegratorSaturationLimit=-inf  POutMin=[]  POutMax=[]  IOutMin=[]  IOutMax=[]  DOutMin=[]  DOutMax=[]  NOutMin=[]  NOutMax=[]  SumOutMin=[]  SumOutMax=[]  SaturationOutMin=[]  SaturationOutMax=[]  PParamMin=[]  PParamMax=[]  IParamMin=[]  IParamMax=[]  DParamMin=[]  DParamMax=[]  NParamMin=[]  NParamMax=[]  KbParamMin=[]  KbParamMax=[]  KtParamMin=[]  KtParamMax=[]  KbOutMin=[]  KbOutMax=[]  KtOutMin=[]  KtOutMax=[]  IntegratorOutMin=[]  IntegratorOutMax=[]  FilterOutMin=[]  FilterOutMax=[]  SumI1OutMin=[]  SumI1OutMax=[]  SumI2OutMin=[]  SumI2OutMax=[]  SumI3OutMin=[]  SumI3OutMax=[]  SumI4OutMin=[]  SumI4OutMax=[]  SumDOutMin=[]  SumDOutMax=[]  DifferentiatorOutMin=[]  DifferentiatorOutMax=[]  FilterDiffOutCoefMin=[]  FilterDiffOutCoefMax=[]  ReciprocalOutMin=[]  ReciprocalOutMax=[]  SumDenOutMin=[]  SumDenOutMax=[]  SumNumOutMin=[]  SumNumOutMax=[]  DivideOutMin=[]  DivideOutMax=[]  UdiffTsProdOutMin=[]  UdiffTsProdOutMax=[]  NTsProdOutMin=[]  NTsProdOutMax=[]  UintegralTsProdOutMin=[]  UintegralTsProdOutMax=[]  UngainTsProdOutMin=[]  UngainTsProdOutMax=[]  ClampingZeroOutDataTypeStr=Inherit: Inherit via back propagation  ClampingZeroOutMin=[]  ClampingZeroOutMax=[]  FilterDenConstantOutDataTypeStr=Inherit: Inherit via back propagation  FilterDenConstantOutMin=[]  FilterDenConstantOutMax=[]  PCopyOutDataTypeStr=Inherit: Inherit via back propagation  PCopyOutMin=[]  PCopyOutMax=[]  NCopyOutDataTypeStr=Inherit: Inherit via back propagation  NCopyOutMin=[]  NCopyOutMax=[]  IntegratorContinuousStateAttributes=''  IntegratorStateMustResolveToSignalObject=off  IntegratorRTWStateStorageClass=Auto  FilterContinuousStateAttributes=''  FilterStateMustResolveToSignalObject=off  FilterRTWStateStorageClass=Auto  ParallelPVariant=InternalParameters  IdealPVariant=Disabled  IVariant=InternalParameters  DVariant=Disabled  IntegratorVariant=Continuous  SatVariant=Enabled  AWVariant=Passthrough  PCopyVariant=Disabled  TRVariant=Disabled  FdbkBlocksVariant=Forward  IdealPFdbkVariant=Disabled  SatFdbkVariant=Disabled  DerivativeFilterVariant=Disabled  NVariant=Disabled  NCopyVariant=Disabled_SignalSpec  FilterICVariant=Disabled  IntegratorICVariant=InternalICs  ExternalResetVariant=Disabled  TRSumVariant=Passthrough  SumFdbkVariant=Disabled  SumVariant=Sum_PI  TsampFilterVariant=InternalTs  TsampNgainVariant=Passthrough  TsampIntegralVariant=Disabled_SignalSpec  ExternalSaturationOutDataTypeStr=Inherit: Same as second input  DerivativeSourceVariant=Disabled  PreIntVariant=InternalPreInt
  Subsystem3 : Subsystem
      settings: PortSchema="{\"entries\":[{\"content\":{\"sides\":[{\"content\":{\"connectorIds\":[\"In1\",\"In2\"]},\"type\":\"ConnectorPlacement.EquallySpacedRectSide\",\"uuid\":\"51b045c8-d819-4b7c-a29d-1a54f5fd995d\"},{\"content\":{\"connectorIds\":[\"Out1\"],\"side\":\"RIGHT\"},\"type\":\"ConnectorPlacement.EquallySpacedRectSide\",\"uuid\":\"9f0647dc-9c35-4883-9e64-6da00897cce8\"},{\"content\":{\"connectorIds\":[\"In3\"],\"side\":\"TOP\"},\"type\":\"ConnectorPlacement.EquallySpacedRectSide\",\"uuid\":\"a4aa7abf-9a58-441d-bef7-3a2aafbde944\"}]},\"type\":\"ConnectorPlacement.EquallySpacedConnector\",\"uuid\":\"237ebc79-3794-4318-8db8-2d16dc313947\"}],\"packageUris\":[\"http://schema.mathworks.com/mf0/Connector/R2020b\"],\"version\":\"1.0\"}"
  Subtract1 : Sum  Inputs=+-
  P : Outport
  wires:
  Meas/1 -> Mean1/1
  Mean1/1 -> Subtract1/2
  Subtract1/1 -> PID Controller1/1
  Ref/1 -> Subtract1/1
  Delay/1 -> Subsystem3/3(Delay)
  PID Controller1/1 -> Subsystem3/1(D)
  Constant2/1 -> Subsystem3/2(P)
  Subsystem3/1(Out) -> P/1

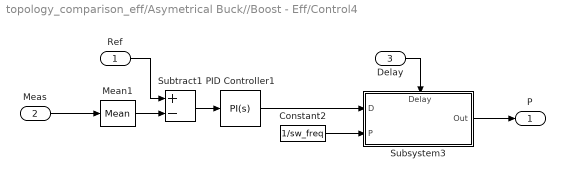
== system topology_comparison_eff/Asymetrical Buck//Boost - Eff/Control4 ==
  Ref : Inport
  Meas : Inport  Port=2
  Delay : Inport  Port=3
  Constant2 : Constant  Value=1/sw_freq
  Mean1 : spsMeanLib/Mean  Freq=sw_freq/10  Vinit=0  Ts=0
  PID Controller1 : slpidlib/PID Controller  Controller=PI  Form=Parallel  TimeDomain=Continuous-time  UseExternalTs=off  SampleTime=-1  IntegratorMethod=Forward Euler  FilterMethod=Forward Euler  ControllerParametersSource=internal  P=asym_bdc_p  I=asym_bdc_i  UseKiTs=on  D=0  UseExternalDerivativeSource=off  N=100  UseFilter=on  TunerSelectOption=Transfer Function Based (PID Tuner App)  InitialConditionSource=internal  InitialConditionForIntegrator=0.18  InitialConditionForFilter=0.1  DifferentiatorICPrevScaledInput=0  ExternalReset=none  TrackingMode=off  Kt=1  LimitOutput=on  SatLimitsSource=internal  UpperSaturationLimit=1  LowerSaturationLimit=0.01  LinearizeAsGain=on  AntiWindupMode=none  Kb=1  LimitIntegrator=off  UpperIntegratorSaturationLimit=inf  LowerIntegratorSaturationLimit=-inf  POutMin=[]  POutMax=[]  IOutMin=[]  IOutMax=[]  DOutMin=[]  DOutMax=[]  NOutMin=[]  NOutMax=[]  SumOutMin=[]  SumOutMax=[]  SaturationOutMin=[]  SaturationOutMax=[]  PParamMin=[]  PParamMax=[]  IParamMin=[]  IParamMax=[]  DParamMin=[]  DParamMax=[]  NParamMin=[]  NParamMax=[]  KbParamMin=[]  KbParamMax=[]  KtParamMin=[]  KtParamMax=[]  KbOutMin=[]  KbOutMax=[]  KtOutMin=[]  KtOutMax=[]  IntegratorOutMin=[]  IntegratorOutMax=[]  FilterOutMin=[]  FilterOutMax=[]  SumI1OutMin=[]  SumI1OutMax=[]  SumI2OutMin=[]  SumI2OutMax=[]  SumI3OutMin=[]  SumI3OutMax=[]  SumI4OutMin=[]  SumI4OutMax=[]  SumDOutMin=[]  SumDOutMax=[]  DifferentiatorOutMin=[]  DifferentiatorOutMax=[]  FilterDiffOutCoefMin=[]  FilterDiffOutCoefMax=[]  ReciprocalOutMin=[]  ReciprocalOutMax=[]  SumDenOutMin=[]  SumDenOutMax=[]  SumNumOutMin=[]  SumNumOutMax=[]  DivideOutMin=[]  DivideOutMax=[]  UdiffTsProdOutMin=[]  UdiffTsProdOutMax=[]  NTsProdOutMin=[]  NTsProdOutMax=[]  UintegralTsProdOutMin=[]  UintegralTsProdOutMax=[]  UngainTsProdOutMin=[]  UngainTsProdOutMax=[]  ClampingZeroOutDataTypeStr=Inherit: Inherit via back propagation  ClampingZeroOutMin=[]  ClampingZeroOutMax=[]  FilterDenConstantOutDataTypeStr=Inherit: Inherit via back propagation  FilterDenConstantOutMin=[]  FilterDenConstantOutMax=[]  PCopyOutDataTypeStr=Inherit: Inherit via back propagation  PCopyOutMin=[]  PCopyOutMax=[]  NCopyOutDataTypeStr=Inherit: Inherit via back propagation  NCopyOutMin=[]  NCopyOutMax=[]  IntegratorContinuousStateAttributes=''  IntegratorStateMustResolveToSignalObject=off  IntegratorRTWStateStorageClass=Auto  FilterContinuousStateAttributes=''  FilterStateMustResolveToSignalObject=off  FilterRTWStateStorageClass=Auto  ParallelPVariant=InternalParameters  IdealPVariant=Disabled  IVariant=InternalParameters  DVariant=Disabled  IntegratorVariant=Continuous  SatVariant=Enabled  AWVariant=Passthrough  PCopyVariant=Disabled  TRVariant=Disabled  FdbkBlocksVariant=Forward  IdealPFdbkVariant=Disabled  SatFdbkVariant=Disabled  DerivativeFilterVariant=Disabled  NVariant=Disabled  NCopyVariant=Disabled_SignalSpec  FilterICVariant=Disabled  IntegratorICVariant=InternalICs  ExternalResetVariant=Disabled  TRSumVariant=Passthrough  SumFdbkVariant=Disabled  SumVariant=Sum_PI  TsampFilterVariant=InternalTs  TsampNgainVariant=Passthrough  TsampIntegralVariant=Disabled_SignalSpec  ExternalSaturationOutDataTypeStr=Inherit: Same as second input  DerivativeSourceVariant=Disabled  PreIntVariant=InternalPreInt
  Subsystem3 : Subsystem
      settings: PortSchema="{\"entries\":[{\"content\":{\"sides\":[{\"content\":{\"connectorIds\":[\"In1\",\"In2\"]},\"type\":\"ConnectorPlacement.EquallySpacedRectSide\",\"uuid\":\"51b045c8-d819-4b7c-a29d-1a54f5fd995d\"},{\"content\":{\"connectorIds\":[\"Out1\"],\"side\":\"RIGHT\"},\"type\":\"ConnectorPlacement.EquallySpacedRectSide\",\"uuid\":\"9f0647dc-9c35-4883-9e64-6da00897cce8\"},{\"content\":{\"connectorIds\":[\"In3\"],\"side\":\"TOP\"},\"type\":\"ConnectorPlacement.EquallySpacedRectSide\",\"uuid\":\"a4aa7abf-9a58-441d-bef7-3a2aafbde944\"}]},\"type\":\"ConnectorPlacement.EquallySpacedConnector\",\"uuid\":\"237ebc79-3794-4318-8db8-2d16dc313947\"}],\"packageUris\":[\"http://schema.mathworks.com/mf0/Connector/R2020b\"],\"version\":\"1.0\"}"
  Subtract1 : Sum  Inputs=+-
  P : Outport
  wires:
  Meas/1 -> Mean1/1
  Mean1/1 -> Subtract1/2
  Subtract1/1 -> PID Controller1/1
  Subsystem3/1(Out) -> P/1
  Ref/1 -> Subtract1/1
  Constant2/1 -> Subsystem3/2(P)
  Delay/1 -> Subsystem3/3(Delay)
  PID Controller1/1 -> Subsystem3/1(D)

== system topology_comparison_eff/Asymetrical Buck//Boost - Eff/Subsystem ==
  Ground : spsGroundLib/Ground  LConnTagsString=a
  Series RLC Branch : spsSeriesRLCBranchLib/Series RLC Branch  LConnTagsString=__new0  RConnTagsString=__new0  BranchType=R  Resistance=1e6  Inductance=1e-3  SetiL0=off  InitialCurrent=0  Capacitance=1e-6  Setx0=off  InitialVoltage=0  Measurements=None
  PD : PMIOPort  Side=Left
  connections:
  Ground/LConn1 -- Series RLC Branch/RConn1
  Series RLC Branch/LConn1 -- PD/RConn1

== system topology_comparison_eff/Asymetrical Buck//Boost - Eff/Subsystem1 ==
  Ground : spsGroundLib/Ground  LConnTagsString=a
  Series RLC Branch : spsSeriesRLCBranchLib/Series RLC Branch  LConnTagsString=__new0  RConnTagsString=__new0  BranchType=R  Resistance=1e6  Inductance=1e-3  SetiL0=off  InitialCurrent=0  Capacitance=1e-6  Setx0=off  InitialVoltage=0  Measurements=None
  PD : PMIOPort  Side=Left
  connections:
  Ground/LConn1 -- Series RLC Branch/RConn1
  Series RLC Branch/LConn1 -- PD/RConn1

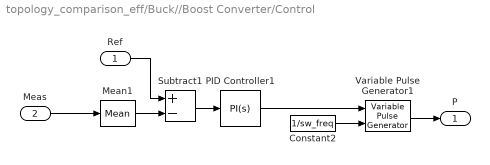
== system topology_comparison_eff/Buck//Boost Converter/Control ==
  Ref : Inport
  Meas : Inport  Port=2
  Constant2 : Constant  Value=1/sw_freq
  Mean1 : spsMeanLib/Mean  Freq=sw_freq/10  Vinit=0  Ts=0
  PID Controller1 : slpidlib/PID Controller  Controller=PI  Form=Parallel  TimeDomain=Continuous-time  UseExternalTs=off  SampleTime=-1  IntegratorMethod=Forward Euler  FilterMethod=Forward Euler  ControllerParametersSource=internal  P=buck_p  I=buck_i  UseKiTs=on  D=0  UseExternalDerivativeSource=off  N=100  UseFilter=on  TunerSelectOption=Transfer Function Based (PID Tuner App)  InitialConditionSource=internal  InitialConditionForIntegrator=0.13  InitialConditionForFilter=0  DifferentiatorICPrevScaledInput=0  ExternalReset=none  TrackingMode=off  Kt=1  LimitOutput=on  SatLimitsSource=internal  UpperSaturationLimit=1  LowerSaturationLimit=0.01  LinearizeAsGain=on  AntiWindupMode=none  Kb=1  LimitIntegrator=off  UpperIntegratorSaturationLimit=inf  LowerIntegratorSaturationLimit=-inf  POutMin=[]  POutMax=[]  IOutMin=[]  IOutMax=[]  DOutMin=[]  DOutMax=[]  NOutMin=[]  NOutMax=[]  SumOutMin=[]  SumOutMax=[]  SaturationOutMin=[]  SaturationOutMax=[]  PParamMin=[]  PParamMax=[]  IParamMin=[]  IParamMax=[]  DParamMin=[]  DParamMax=[]  NParamMin=[]  NParamMax=[]  KbParamMin=[]  KbParamMax=[]  KtParamMin=[]  KtParamMax=[]  KbOutMin=[]  KbOutMax=[]  KtOutMin=[]  KtOutMax=[]  IntegratorOutMin=[]  IntegratorOutMax=[]  FilterOutMin=[]  FilterOutMax=[]  SumI1OutMin=[]  SumI1OutMax=[]  SumI2OutMin=[]  SumI2OutMax=[]  SumI3OutMin=[]  SumI3OutMax=[]  SumI4OutMin=[]  SumI4OutMax=[]  SumDOutMin=[]  SumDOutMax=[]  DifferentiatorOutMin=[]  DifferentiatorOutMax=[]  FilterDiffOutCoefMin=[]  FilterDiffOutCoefMax=[]  ReciprocalOutMin=[]  ReciprocalOutMax=[]  SumDenOutMin=[]  SumDenOutMax=[]  SumNumOutMin=[]  SumNumOutMax=[]  DivideOutMin=[]  DivideOutMax=[]  UdiffTsProdOutMin=[]  UdiffTsProdOutMax=[]  NTsProdOutMin=[]  NTsProdOutMax=[]  UintegralTsProdOutMin=[]  UintegralTsProdOutMax=[]  UngainTsProdOutMin=[]  UngainTsProdOutMax=[]  ClampingZeroOutDataTypeStr=Inherit: Inherit via back propagation  ClampingZeroOutMin=[]  ClampingZeroOutMax=[]  FilterDenConstantOutDataTypeStr=Inherit: Inherit via back propagation  FilterDenConstantOutMin=[]  FilterDenConstantOutMax=[]  PCopyOutDataTypeStr=Inherit: Inherit via back propagation  PCopyOutMin=[]  PCopyOutMax=[]  NCopyOutDataTypeStr=Inherit: Inherit via back propagation  NCopyOutMin=[]  NCopyOutMax=[]  IntegratorContinuousStateAttributes=''  IntegratorStateMustResolveToSignalObject=off  IntegratorRTWStateStorageClass=Auto  FilterContinuousStateAttributes=''  FilterStateMustResolveToSignalObject=off  FilterRTWStateStorageClass=Auto  ParallelPVariant=InternalParameters  IdealPVariant=Disabled  IVariant=InternalParameters  DVariant=Disabled  IntegratorVariant=Continuous  SatVariant=Enabled  AWVariant=Passthrough  PCopyVariant=Disabled  TRVariant=Disabled  FdbkBlocksVariant=Forward  IdealPFdbkVariant=Disabled  SatFdbkVariant=Disabled  DerivativeFilterVariant=Disabled  NVariant=Disabled  NCopyVariant=Disabled_SignalSpec  FilterICVariant=Disabled  IntegratorICVariant=InternalICs  ExternalResetVariant=Disabled  TRSumVariant=Passthrough  SumFdbkVariant=Disabled  SumVariant=Sum_PI  TsampFilterVariant=InternalTs  TsampNgainVariant=Passthrough  TsampIntegralVariant=Disabled_SignalSpec  ExternalSaturationOutDataTypeStr=Inherit: Same as second input  DerivativeSourceVariant=Disabled  PreIntVariant=InternalPreInt
  Subtract1 : Sum  Inputs=+-
  Variable Pulse Generator1 : VariablePulseGenerator  AllowZeroPulseWidth=on  SampleTime=0.1
  P : Outport
  wires:
  Meas/1 -> Mean1/1
  PID Controller1/1 -> Variable Pulse Generator1/1
  Constant2/1 -> Variable Pulse Generator1/2
  Mean1/1 -> Subtract1/2
  Subtract1/1 -> PID Controller1/1
  Variable Pulse Generator1/1 -> P/1
  Ref/1 -> Subtract1/1
